simulink model "game2022a"  (R2022a)
settings: Solver=VariableStepAuto  StartTime=0.0  StopTime=Inf  RelTol=1e-3
libraries: robotlib x6
settings Model: Creator=michaelnaps  LastModifiedBy=michaelnaps
settings ModelReferenceCC: EnableRefExpFcnMdlSchedulingChecks=off
settings RTWCC: Description=Generic Real-Time Target

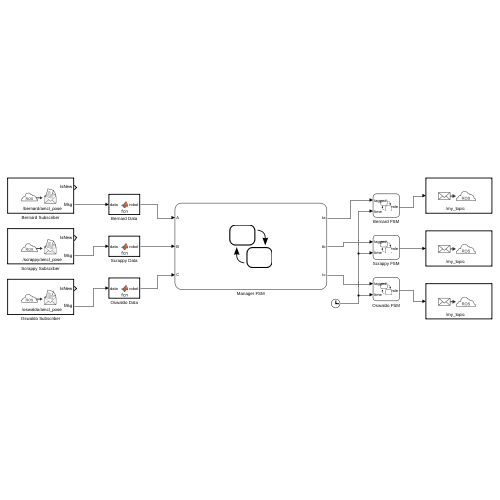
[thumbnail: Simulink's stored preview of the top-level diagram]
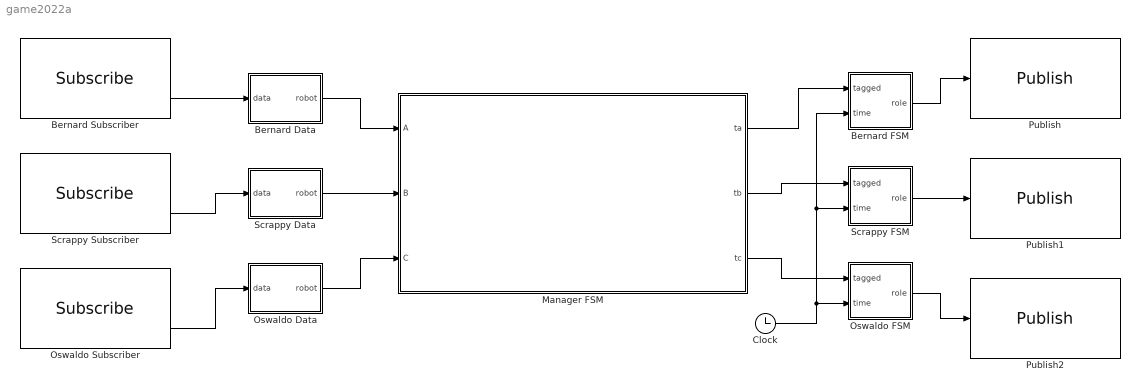
== system game2022a ==
  Bernard Data : MATLAB Function  TreatAsAtomicUnit=on
  Bernard FSM : Stateflow chart  TreatAsAtomicUnit=on
  Bernard Subscriber : robotlib/Subscribe  topicSource=Select from ROS network  topic=/bernard/amcl_pose  messageType=geometry_msgs/PoseWithCovarianceStamped  SampleTime=-1  legacyBusStruct=off  messageQueueLength=1
  Clock : Clock
  Manager FSM : Stateflow chart  TreatAsAtomicUnit=on
  Oswaldo Data : MATLAB Function  TreatAsAtomicUnit=on
  Oswaldo FSM : Stateflow chart  TreatAsAtomicUnit=on
  Oswaldo Subscriber : robotlib/Subscribe  topicSource=Specify your own  topic=/oswaldo/amcl_pose  messageType=geometry_msgs/Point  SampleTime=-1  legacyBusStruct=off  messageQueueLength=1
  Publish : robotlib/Publish  topicSource=Select from ROS network  topic=/my_topic  messageType=geometry_msgs/Point  legacyBusStruct=off  messageQueueLength=1
  Publish1 : robotlib/Publish  topicSource=Select from ROS network  topic=/my_topic  messageType=geometry_msgs/Point  legacyBusStruct=off  messageQueueLength=1
  Publish2 : robotlib/Publish  topicSource=Select from ROS network  topic=/my_topic  messageType=geometry_msgs/Point  legacyBusStruct=off  messageQueueLength=1
  Scrappy Data : MATLAB Function  TreatAsAtomicUnit=on
  Scrappy FSM : Stateflow chart  TreatAsAtomicUnit=on
  Scrappy Subscriber : robotlib/Subscribe  topicSource=Select from ROS network  topic=/scrappy/amcl_pose  messageType=geometry_msgs/PoseWithCovarianceStamped  SampleTime=-1  legacyBusStruct=off  messageQueueLength=1
  wires:
  Bernard Subscriber/2 -> Bernard Data/1(data)
  Bernard Data/1(robot) -> Manager FSM/1(A)
  Manager FSM/1(ta) -> Bernard FSM/1(tagged)
  Scrappy Data/1(robot) -> Manager FSM/2(B)
  Oswaldo Data/1(robot) -> Manager FSM/3(C)
  Manager FSM/3(tc) -> Oswaldo FSM/1(tagged)
  Manager FSM/2(tb) -> Scrappy FSM/1(tagged)
  Oswaldo Subscriber/2 -> Oswaldo Data/1(data)
  Scrappy Subscriber/2 -> Scrappy Data/1(data)
  Oswaldo FSM/1(role) -> Publish2/1
  Scrappy FSM/1(role) -> Publish1/1
  Bernard FSM/1(role) -> Publish/1
  Clock/1 -> Oswaldo FSM/2(time), Scrappy FSM/2(time), Bernard FSM/2(time)

== matlab function game2022a/Scrappy Data ==
  data: data input; robot output
function robot = fcn(data)
    robot = data;
end

== matlab function game2022a/Oswaldo Data ==
  data: data input; robot output
function robot = fcn(data)
    robot = data;
end

== stateflow chart game2022a/Bernard FSM ==
  state S_pursuer
    role = "pursuer"
  state S_evader
    role = "evader"
  state S_delay
    role = "paused"
  (default) -> S_pursuer
  S_pursuer -> S_evader : [tagged]
  S_delay -> S_pursuer [order 1] : [(time - p_start) < T]
  S_evader -> S_delay : [tagged]{p_start = time}
  S_delay -> S_delay [order 2] : [(time - p_start) < T]
  data: tagged input; role output; time input double =get_param(bdroot,'FixedStep'); T constant double =1; p_start local

== matlab function game2022a/Bernard Data ==
  data: data input; robot output
function robot = fcn(data)

    disp(data);
    robot = data;
    
end

== stateflow chart game2022a/Manager FSM ==
  state S_ABC
    ta = 0;
    tb = 0;
    tc = 0;
  state S_BAC
    ta = 0;
    tb = 0;
    tc = 0;
  state S_CAB
    ta = 0;
    tb = 0;
    tc = 0;
  (default) -> S_ABC
  S_ABC -> S_BAC [order 1] : [d(A,B) <= W]{ta = 1, tb = 1}
  S_BAC -> S_ABC [order 2] : [d(B,A) <= W]{ta = 1, tb = 1}
  S_ABC -> S_CAB [order 2] : [d(C,A) <= W]{ta = 1, tc = 1}
  S_CAB -> S_ABC [order 2] : [d(C,A) <= W]{ta = 1, tc = 1}
  S_CAB -> S_BAC [order 1] : [d(C,B) <= W]{tb = 1, tc = 1}
  S_BAC -> S_CAB [order 1] : [d(B,C) <= W]{tb = 1, tc = 1}
  data: d constant double; ta output; tb output; tc output; A input; B input; C input; W constant double =tag_radius

== stateflow chart game2022a/Scrappy FSM ==
  state S_pursuer
    role = "pursuer"
  state S_evader
    role = "evader"
  state S_delay
    role = "paused"
  (default) -> S_pursuer
  S_pursuer -> S_evader : [tagged]
  S_delay -> S_pursuer [order 1] : [(time - p_start) < T]
  S_evader -> S_delay : [tagged]{p_start = time}
  S_delay -> S_delay [order 2] : [(time - p_start) < T]
  data: tagged input; role output; T constant double =1; p_start local; time input

== stateflow chart game2022a/Oswaldo FSM ==
  state S_pursuer
    role = "pursuer"
  state S_evader
    role = "evader"
  state S_delay
    role = "paused"
  (default) -> S_pursuer
  S_pursuer -> S_evader : [tagged]
  S_delay -> S_pursuer [order 1] : [(time - p_start) < T]
  S_evader -> S_delay : [tagged]{p_start = time}
  S_delay -> S_delay [order 2] : [(time - p_start) < T]
  data: tagged input; role output; T constant double; p_start local; time input
